simulink model "Two_Modeelling_of_Tn_lines_using_Labels"  (R2024a)
settings: Solver=ode23tb  StartTime=0.0  StopTime=1  MaxStep=1e-4  RelTol=1e-3
libraries: spsRMSLib x8, spsPower3phInstantaneousLib x2, spsThreePhaseVIMeasurementLib x2, spsThreePhaseSeriesRLCBranchLib x1, spsThreePhaseSourceLib x1, spsThreePhaseSeriesRLCLoadLib x1, sps_lib x1
settings Model: Creator=91889  LastModifiedBy=91889

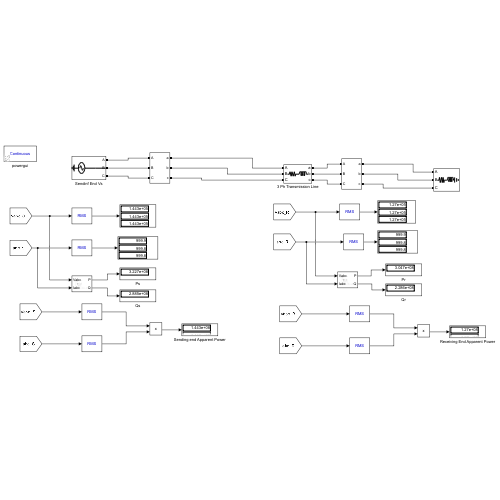
[thumbnail: Simulink's stored preview of the top-level diagram]
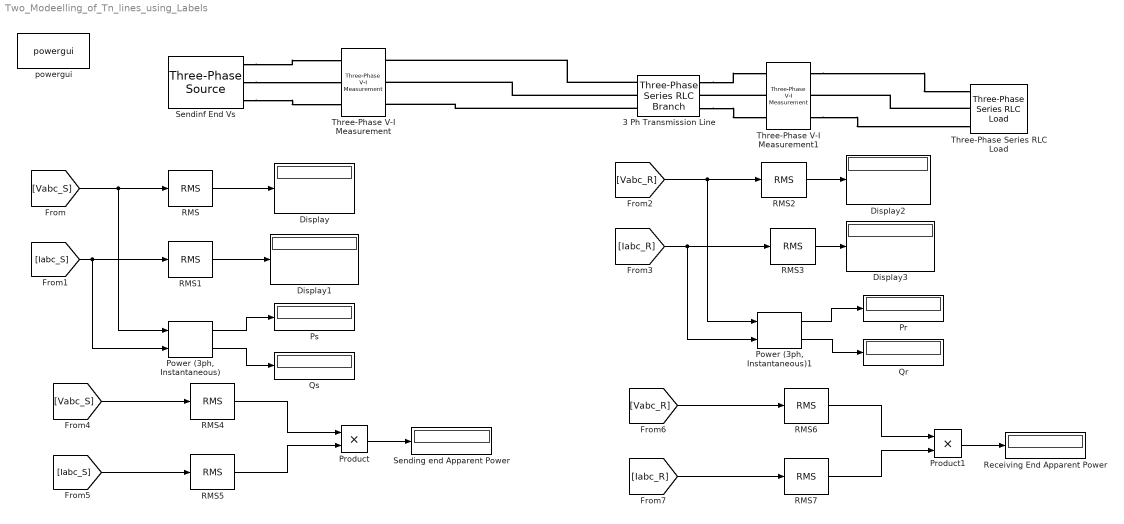
== system Two_Modeelling_of_Tn_lines_using_Labels ==
  3 Ph Transmission Line : spsThreePhaseSeriesRLCBranchLib/Three-Phase Series RLC Branch  LConnTagsString=A|B|C  RConnTagsString=A|B|C  BranchType=RL  Resistance=6  Inductance=0.053052  Capacitance=1e-6  Measurements=None
  Display{,1..3} (4 alike) : Display
  "Power (3ph, Instantaneous)" : spsPower3phInstantaneousLib/Power (3ph, Instantaneous)
  "Power (3ph, Instantaneous)1" : spsPower3phInstantaneousLib/Power (3ph, Instantaneous)
  Pr : Display
  Product : Product
  Product1 : Product
  Ps : Display
  Qr : Display
  Qs : Display
  RMS{,1..7} (8 alike) : spsRMSLib/RMS  TrueRMS=on  Freq=60  RMSInit=0  Ts=0
  Receiving End Apparent Power : Display
  Sendinf End Vs : spsThreePhaseSourceLib/Three-Phase Source  InternalConnection=Yg  VoltagePhases=off  Voltage=250e3  PhaseAngle=0  Voltage_phases=[25e3 25e3 25e3]/sqrt(3)  PhaseAngles_phases=[0 -120 +120]  Frequency=60  NonIdealSource=on  SpecifyImpedance=off  Resistance=0  Inductance=0  ShortCircuitLevel=100e6  BaseVoltage=250e3  XRratio=7  BusType=swing  Pref=10e3  Qref=0  Prefabc=[10e3, 10e3, 10e3]  Qrefabc=[0, 0, 0]  Qmin=-inf  Qmax=inf
  Sending end Apparent Power : Display
  Three-Phase Series RLC Load : spsThreePhaseSeriesRLCLoadLib/Three-Phase Series RLC Load  LConnTagsString=A|B|C  Configuration=Y (grounded)  NominalVoltage=220e3  Vabc=[1e3 1e3 1e3]  Vabcp=[1e3 1e3 1e3]  NominalFrequency=60  UnbalancedPower=off  ActivePower=304.8e6  InductivePower=228.6e6  CapacitivePower=0  Pabc=[10e3 9e3 11e3]  QLabc=[100 90 110]  QCabc=[100 90 110]  Pabcp=[10e3 9e3 11e3]  QLabcp=[100 90 110]  QCabcp=[100 90 110]  Measurements=None  LoadType=constant Z
  Three-Phase V-I Measurement : spsThreePhaseVIMeasurementLib/Three-Phase V-I Measurement  VoltageMeasurement=phase-to-ground  SetLabelV=on  LabelV=Vabc_S  Vpu=off  VpuLL=off  CurrentMeasurement=yes  SetLabelI=on  LabelI=Iabc_S  Ipu=off  Pbase=100e6  Vbase=500e3  OutputType=Complex  PhasorSimulation=off  PSBequivalent=0
  Three-Phase V-I Measurement1 : spsThreePhaseVIMeasurementLib/Three-Phase V-I Measurement  VoltageMeasurement=phase-to-ground  SetLabelV=on  LabelV=Vabc_R  Vpu=off  VpuLL=off  CurrentMeasurement=yes  SetLabelI=on  LabelI=Iabc_R  Ipu=off  Pbase=100e6  Vbase=500e3  OutputType=Complex  PhasorSimulation=off  PSBequivalent=0
  powergui : sps_lib/powergui  Priority=1  SimulationMode=Continuous  SampleTime=50e-6  frequency=60  Iterations=50  frequencyindice=60  Pbase=100e6  ErrMax=1e-4  UnitsV=kV  UnitsW=MW  buscounter=0  FunctionMessages=off  echomessages=off  EnableUseOfTLC=off  CurrentSourceSwitches=off  DisableSnubberDevices=off  DisableRonSwitches=off  DisableVfSwitches=off  DisplayEquations=off  AutomaticDiscreteSolvers=off  SolverType=Tustin/Backward Euler (TBE)  Interpol=off  ExternalGateDelay=off  methode=off  Ts=100  x0status=blocks  SPID=on  SwTol=0  HookPort=off  NonlinearTolerance=1e-4  nMaxIteration=100  ContinueOnMaxIteration=off  RestoreLinks=warning  ResistiveCurrentMeasurement=off  Frange=[0:2:500]  Ylog=off  Xlog=on  ShowGrid=off  save=off  variable=ZData  structure=0  ZoomFFT=off  StartTime=0.0  cycles=1  DisplayStyle=1  fundamental=60  FreqAxis=off  MaxFrequency=1000  frequencyindicesteady=1  RmsSteady=1  display=off
  wires:
  [Vabc_S] -> "Power (3ph, Instantaneous)"/1, RMS/1
  RMS/1 -> Display/1
  [Iabc_S] -> "Power (3ph, Instantaneous)"/2, RMS1/1
  RMS1/1 -> Display1/1
  RMS2/1 -> Display2/1
  RMS3/1 -> Display3/1
  "Power (3ph, Instantaneous)"/1 -> Ps/1
  "Power (3ph, Instantaneous)"/2 -> Qs/1
  "Power (3ph, Instantaneous)1"/1 -> Pr/1
  [Iabc_R] -> "Power (3ph, Instantaneous)1"/2, RMS3/1
  "Power (3ph, Instantaneous)1"/2 -> Qr/1
  [Vabc_R] -> "Power (3ph, Instantaneous)1"/1, RMS2/1
  RMS4/1 -> Product/1
  [Iabc_S] -> RMS5/1
  RMS5/1 -> Product/2
  [Vabc_S] -> RMS4/1
  Product/1 -> Sending end Apparent Power/1
  RMS7/1 -> Product1/2
  [Iabc_R] -> RMS7/1
  Product1/1 -> Receiving End Apparent Power/1
  [Vabc_R] -> RMS6/1
  RMS6/1 -> Product1/1
  connections:
  Three-Phase V-I Measurement1/RConn3 -- Three-Phase Series RLC Load/LConn3
  Sendinf End Vs/RConn2 -- Three-Phase V-I Measurement/LConn2
  Sendinf End Vs/RConn1 -- Three-Phase V-I Measurement/LConn1
  3 Ph Transmission Line/RConn1 -- Three-Phase V-I Measurement1/LConn1
  Sendinf End Vs/RConn3 -- Three-Phase V-I Measurement/LConn3
  3 Ph Transmission Line/LConn1 -- Three-Phase V-I Measurement/RConn1
  3 Ph Transmission Line/LConn2 -- Three-Phase V-I Measurement/RConn2
  Three-Phase V-I Measurement1/RConn1 -- Three-Phase Series RLC Load/LConn1
  Three-Phase V-I Measurement1/LConn2 -- 3 Ph Transmission Line/RConn2
  3 Ph Transmission Line/LConn3 -- Three-Phase V-I Measurement/RConn3
  Three-Phase Series RLC Load/LConn2 -- Three-Phase V-I Measurement1/RConn2
  3 Ph Transmission Line/RConn3 -- Three-Phase V-I Measurement1/LConn3
